simulink library "xrbsDSP_r3"  (Simulink 5.0)
undefined symbols (not defined in the file or in its folder): FIR1, Ft, mem
libraries: xbsIndex_r3 x329
(part 2 of 4)

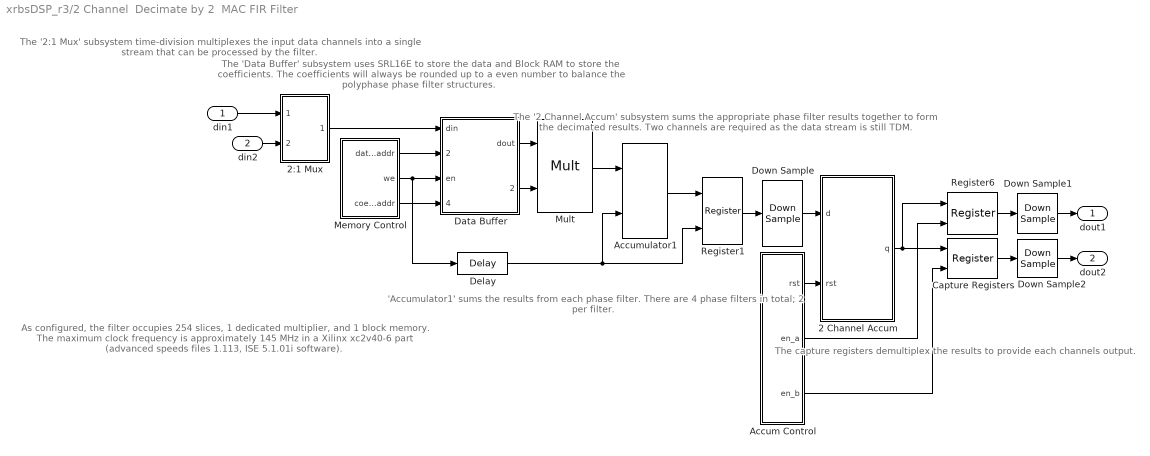
== system xrbsDSP_r3/2 Channel  Decimate by 2  MAC FIR Filter ==
  note: As configured, the  filter occupies 254 slices, 1 dedicated multiplier, and
      | 1 block memory.  The maximum clock frequency is approximately
      | 145 MHz in a Xilinx xc2v40-6 part (advanced speeds files 1.113, ISE
      | 5.1.01i software).
  note: The capture registers demultiplex
      | the results to provide each
      | channels output.
  note: The '2 Channel Accum' subsystem sums the
      | appropriate phase filter results together to
      | form the decimated results.  Two channels
      | are required as the data stream is still TDM.
  note: 'Accumulator1' sums the results
      | from each phase filter.  There
      | are 4 phase filters in total; 2 per
      | filter.
  note: The 'Data Buffer' subsystem uses SRL16E to store
      | the data and Block RAM to store the
      | coefficients. The coefficients will always
      | be rounded up to a even number to balance the
      | polyphase phase filter structures.
  note: The '2:1 Mux' subsystem time-division
      | multiplexes the input data channels
      | into a single stream that can be
      | processed by the filter.
  din1 : Inport
  din2 : Inport  Port=2
  2 Channel Accum : Subsystem
  2:1 Mux : Subsystem
  Accum Control : Subsystem
  Accumulator1 : xbsIndex_r3/Accumulator  n_bits=accum2_bit_width  overflow=Wrap  operation=Add  scale=1  explicit_period=off  period=1  rst=on  hasbypass=on  en=off  dbl_ovrd=off  show_param=off  gen_core=on  use_rpm=off
      settings: xl_area=[0, 0, 0, 0, 0, 0, 0]
  Capture Registers : xbsIndex_r3/Register  init=0  reg_only_valid=off  explicit_period=off  period=1  rst=off  en=on  out_en=on  dbl_ovrd=off  show_param=off
      settings: xl_area=[0, 0, 0, 0, 0, 0, 0]
  Data Buffer : Subsystem
  Delay : xbsIndex_r3/Delay  latency=4  reg_retiming=off  explicit_period=off  period=1  en=off  accept_only_valid=off  init_zero=on  dbl_ovrd=off  show_param=off
      settings: xl_area=[0, 0, 0, 0, 0, 0, 0]
  Down Sample : xbsIndex_r3/Down Sample  sample_ratio=length(coef)/4  sample_phase="Last Value of Frame  (most efficient)"  latency=1  en=off  dbl_ovrd=off  show_param=off
      settings: xl_area=[0, 0, 0, 0, 0, 0, 0]
  Down Sample1 : xbsIndex_r3/Down Sample  sample_ratio=4  sample_phase="Last Value of Frame  (most efficient)"  latency=1  en=off  dbl_ovrd=off  show_param=off
      settings: xl_area=[19 37 0 0 0 0 0]
  Down Sample2 : xbsIndex_r3/Down Sample  sample_ratio=4  sample_phase="Last Value of Frame  (most efficient)"  latency=1  en=off  dbl_ovrd=off  show_param=off
      settings: xl_area=[19 37 0 0 0 0 0]
  Memory Control : Subsystem
  Mult : xbsIndex_r3/Mult  precision=Full  arith_type="Signed  (2's comp)"  n_bits=8  bin_pt=2  quantization=Truncate  overflow=Wrap  latency=2  explicit_period=off  period=1  en=off  dbl_ovrd=off  show_param=off  mult_type=Parallel  oversample=2  use_embedded=on  pipeline=on  use_rpm=off  placement_style=Rectangular Shape  gen_core=on
      settings: xl_area=[0, 0, 0, 0, 0, 0, 0]
  Register1 : xbsIndex_r3/Register  init=0  reg_only_valid=off  explicit_period=off  period=1  rst=off  en=on  out_en=off  dbl_ovrd=off  show_param=off
      settings: xl_area=[0, 0, 0, 0, 0, 0, 0]
  Register6 : xbsIndex_r3/Register  init=0  reg_only_valid=off  explicit_period=off  period=1  rst=off  en=on  out_en=on  dbl_ovrd=off  show_param=off
      settings: xl_area=[0, 0, 0, 0, 0, 0, 0]
  dout1 : Outport
  dout2 : Outport  Port=2
  wires:
  Down Sample2/1 -> dout2/1
  Down Sample1/1 -> dout1/1
  Down Sample/1 -> 2 Channel Accum/1(d)
  din2/1 -> 2:1 Mux/2(din2)
  Accum Control/3(en_b) -> Capture Registers/2
  Accum Control/2(en_a) -> Register6/2
  Accum Control/1(rst) -> 2 Channel Accum/2(rst)
  Capture Registers/1 -> Down Sample2/1
  2 Channel Accum/1(q) -> Register6/1, Capture Registers/1
  Register6/1 -> Down Sample1/1
  Accumulator1/1 -> Register1/1
  Memory Control/3(coef_addr) -> Data Buffer/4(coef_addr)
  Memory Control/2(we) -> Delay/1, Data Buffer/3(en)
  Memory Control/1(data_addr) -> Data Buffer/2(data_addr)
  Data Buffer/1(dout) -> Mult/1
  Mult/1 -> Accumulator1/1
  Delay/1 -> Accumulator1/2, Register1/2
  Register1/1 -> Down Sample/1
  Data Buffer/2(coef_out) -> Mult/2
  2:1 Mux/1(dout) -> Data Buffer/1(din)
  din1/1 -> 2:1 Mux/1(din1)

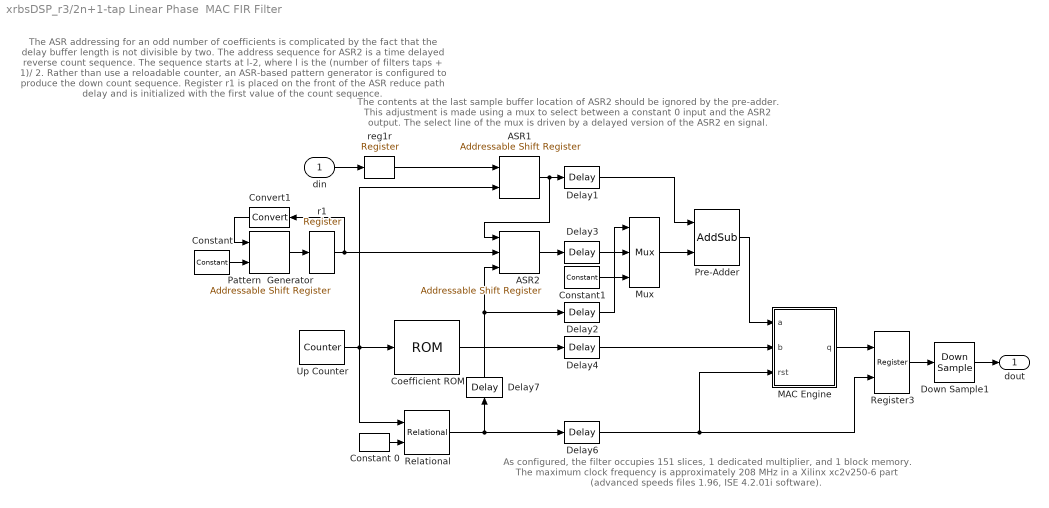
== system xrbsDSP_r3/2n+1-tap Linear Phase  MAC FIR Filter ==
  note: The ASR addressing for an odd number of coefficients is
      | complicated by the fact that the delay buffer length is not
      | divisible by two.  The address sequence for ASR2 is a time
      | delayed reverse count sequence.  The sequence starts at
      | l-2,  where l is the (number of filters taps + 1)/ 2.  Rather
      | than use a reloadable counter, an ASR-based pattern
      | generator is configured to produce the down count
      | sequence.  Register r1 is placed on the front of the ASR
      | reduce path delay and is initialized with the first value of
      | the count sequence.
  note: The contents at the last sample buffer location
      | of ASR2 should be ignored by the pre-adder.
      | This adjustment is made using a mux to select
      | between a constant 0 input and the ASR2 output.
      | The select line of the mux is driven by a delayed
      | version of the ASR2 en signal.
  note: As configured, the  filter occupies 151 slices, 1 dedicated multiplier, and
      | 1 block memory.  The maximum clock frequency is approximately
      | 208 MHz in a Xilinx xc2v250-6 part (advanced speeds files 1.96, ISE
      | 4.2.01i software).
  din : Inport
  ASR1 : xbsIndex_r3/Addressable Shift Register  infer_latency=on  depth=2  initVector=0  explicit_period=off  period=1  accept_only_valid=off  en=off  dbl_ovrd=off  show_param=off  use_rpm=off  gen_core=off
      settings: xl_area=[0, 0, 0, 0, 0, 0, 0]
  ASR2 : xbsIndex_r3/Addressable Shift Register  infer_latency=on  depth=2  initVector=0  explicit_period=off  period=1  accept_only_valid=off  en=on  dbl_ovrd=off  show_param=off  use_rpm=off  gen_core=off
      settings: xl_area=[0, 0, 0, 0, 0, 0, 0]
  Coefficient ROM : xbsIndex_r3/ROM  depth=(length(coef)+1)/2  initVector=coef(1:((length(coef)+1)/2))  arith_type="Signed  (2's comp)"  n_bits=coef_n_bits  bin_pt=coef_bin_pt  latency=1  init_zero=on  explicit_period=off  period=1  rst=off  init_reg=0  en=off  dbl_ovrd=off  show_param=off  distributed_mem=off  use_rpm=off  gen_core=on
      settings: xl_area=[0, 0, 0, 0, 0, 0, 0]
  Constant : xbsIndex_r3/Constant  const=(length(coef)+1)/2-2  arith_type=Unsigned  n_bits=ceil(log2(((length(coef)+1)/2-1)))  bin_pt=0  explicit_period=on  period=smpl_period/((length(coef)+1)/2)  dbl_ovrd=off
  Constant 0 : xbsIndex_r3/Constant  const=0  arith_type=Unsigned  n_bits=1  bin_pt=0  explicit_period=off  period=1  dbl_ovrd=off
  Constant1 : xbsIndex_r3/Constant  const=0  arith_type=Unsigned  n_bits=1  bin_pt=0  explicit_period=off  period=1  dbl_ovrd=off
  Convert1 : xbsIndex_r3/Convert  Orientation=left  arith_type=Unsigned  n_bits=ceil(log2((length(coef)+1)/2))  bin_pt=0  quantization=Truncate  overflow=Wrap  latency=0  explicit_period=off  period=1  dbl_ovrd=off  show_param=off  inserted_by_tool=off
      settings: xl_area=[0, 0, 0, 0, 0, 0, 0]
  Delay1 : xbsIndex_r3/Delay  latency=2  reg_retiming=off  explicit_period=off  period=1  en=off  accept_only_valid=off  init_zero=on  dbl_ovrd=off  show_param=off
      settings: xl_area=[0, 0, 0, 0, 0, 0, 0]
  Delay2 : xbsIndex_r3/Delay  latency=1  reg_retiming=off  explicit_period=off  period=1  en=off  accept_only_valid=off  init_zero=on  dbl_ovrd=off  show_param=off
      settings: xl_area=[0, 0, 0, 0, 0, 0, 0]
  Delay3 : xbsIndex_r3/Delay  latency=1  reg_retiming=off  explicit_period=off  period=1  en=off  accept_only_valid=off  init_zero=on  dbl_ovrd=off  show_param=off
      settings: xl_area=[0, 0, 0, 0, 0, 0, 0]
  Delay4 : xbsIndex_r3/Delay  latency=2  reg_retiming=off  explicit_period=off  period=1  en=off  accept_only_valid=off  init_zero=on  dbl_ovrd=off  show_param=off
      settings: xl_area=[0, 0, 0, 0, 0, 0, 0]
  Delay6 : xbsIndex_r3/Delay  latency=4  reg_retiming=off  explicit_period=off  period=1  en=off  accept_only_valid=off  init_zero=on  dbl_ovrd=off  show_param=off
      settings: xl_area=[0, 0, 0, 0, 0, 0, 0]
  Delay7 : xbsIndex_r3/Delay  Orientation=up  latency=((length(coef)+1)/2)-2  reg_retiming=off  explicit_period=off  period=1  en=off  accept_only_valid=off  init_zero=on  dbl_ovrd=off  show_param=off
      settings: xl_area=[0, 0, 0, 0, 0, 0, 0]
  Down Sample1 : xbsIndex_r3/Down Sample  sample_ratio=(length(coef)+1)/2  sample_phase="Last Value of Frame  (most efficient)"  latency=1  en=off  dbl_ovrd=off  show_param=off
      settings: xl_area=[0, 0, 0, 0, 0, 0, 0]
  MAC Engine : Subsystem
  Mux : xbsIndex_r3/Mux  inputs=2  precision=Full  arith_type="Signed  (2's comp)"  n_bits=8  bin_pt=2  quantization=Truncate  overflow=Wrap  latency=1  explicit_period=off  period=1  en=off  dbl_ovrd=off  show_param=off  mux_type=off  use_rpm=off  gen_core=on
      settings: xl_area=[0, 0, 0, 0, 0, 0, 0]
  Pattern  Generator : xbsIndex_r3/Addressable Shift Register  infer_latency=on  depth=2  initVector=[((length(coef)+1)/2)-1 (0:(length(coef)+1)/2-3)]  explicit_period=off  period=1  accept_only_valid=off  en=off  dbl_ovrd=off  show_param=off  use_rpm=off  gen_core=off
      settings: xl_area=[0, 0, 0, 0, 0, 0, 0]
  Pre-Adder : xbsIndex_r3/AddSub  mode=Addition  precision=Full  arith_type=Unsigned  n_bits=8  bin_pt=2  quantization=Truncate  overflow=Wrap  latency=1  explicit_period=off  period=1  use_carryin=off  use_carryout=off  en=off  dbl_ovrd=off  show_param=off  use_core=on  pipeline=off  use_rpm=off  gen_core=on
      settings: xl_area=[0, 0, 0, 0, 0, 0, 0]
  Register3 : xbsIndex_r3/Register  init=0  reg_only_valid=on  explicit_period=off  period=1  rst=off  en=on  out_en=off  dbl_ovrd=off  show_param=off
      settings: xl_area=[0, 0, 0, 0, 0, 0, 0]
  Relational : xbsIndex_r3/Relational  mode=a=b  latency=1  explicit_period=off  period=1  en=off  dbl_ovrd=off  show_param=off
      settings: xl_area=[0, 0, 0, 0, 0, 0, 0]
  Up Counter : xbsIndex_r3/Counter  cnt_type=Count Limited  n_bits=ceil(log2((length(coef)+1)/2))  bin_pt=0  arith_type=Unsigned  start_count=0  cnt_to=((length(coef)+1)/2)-1  cnt_by_val=1  operation=Up  explicit_period=on  period=smpl_period/((length(coef)+1)/2)  load_pin=off  rst=off  en=off  dbl_ovrd=off  show_param=off  use_rpm=on  gen_core=on
      settings: xl_area=[0, 0, 0, 0, 0, 0, 0]
  r1 : xbsIndex_r3/Register  init=((length(coef)+1)/2)-2  reg_only_valid=off  explicit_period=on  period=smpl_period/((length(coef)+1)/2)  rst=off  en=off  out_en=off  dbl_ovrd=off  show_param=off
      settings: xl_area=[0, 0, 0, 0, 0, 0, 0]
  reg1r : xbsIndex_r3/Register  init=0  reg_only_valid=on  explicit_period=off  period=1  rst=off  en=off  out_en=off  dbl_ovrd=off  show_param=off
      settings: xl_area=[0, 0, 0, 0, 0, 0, 0]
  dout : Outport
  wires:
  Coefficient ROM/1 -> Delay4/1
  Relational/1 -> Delay6/1, Delay7/1
  Constant 0/1 -> Relational/2
  Down Sample1/1 -> dout/1
  din/1 -> reg1r/1
  Up Counter/1 -> Relational/1, Coefficient ROM/1, ASR1/2
  ASR1/1 -> ASR2/1, Delay1/1
  reg1r/1 -> ASR1/1
  Delay1/1 -> Pre-Adder/1
  MAC Engine/1(q) -> Register3/1
  Register3/1 -> Down Sample1/1
  Pre-Adder/1 -> MAC Engine/1(a)
  Delay4/1 -> MAC Engine/2(b)
  Delay6/1 -> Register3/2, MAC Engine/3(rst)
  ASR2/1 -> Delay3/1
  Delay3/1 -> Mux/2
  Pattern  Generator/1 -> r1/1
  Constant/1 -> Pattern  Generator/2
  Convert1/1 -> Pattern  Generator/1
  Mux/1 -> Pre-Adder/2
  Constant1/1 -> Mux/3
  r1/1 -> ASR2/2, Convert1/1
  Delay7/1 -> Delay2/1, ASR2/3
  Delay2/1 -> Mux/1

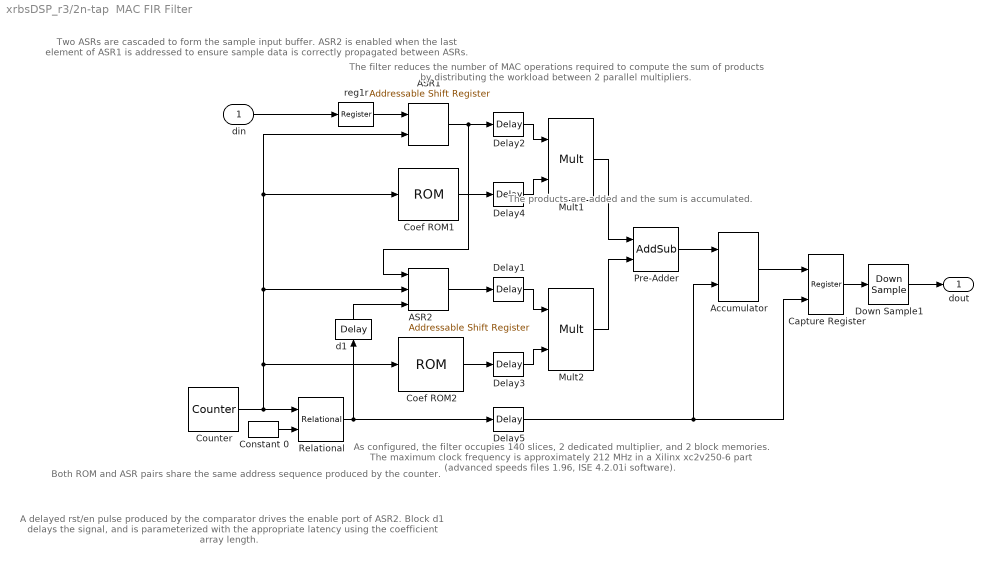
== system xrbsDSP_r3/2n-tap  MAC FIR Filter ==
  note: The filter reduces the number of MAC operations required
      | to compute the sum of products by distributing the workload
      | between 2 parallel multipliers.
  note: Both ROM and ASR pairs share the same
      | address sequence produced by the counter.
  note: The products are added and
      | the sum is accumulated.
  note: As configured, the  filter occupies 140 slices, 2 dedicated multiplier, and
      | 2 block memories.  The maximum clock frequency is approximately
      | 212 MHz in a Xilinx xc2v250-6 part (advanced speeds files 1.96, ISE
      | 4.2.01i software).
  note: Two ASRs are cascaded to form the sample
      | input  buffer.  ASR2 is enabled when the last
      | element of ASR1 is addressed to ensure sample
      | data is correctly propagated between ASRs.
  note: A delayed rst/en pulse produced by the comparator
      | drives the enable port of ASR2.  Block d1 delays the
      | signal, and is parameterized with the appropriate
      | latency using the coefficient array length.
  din : Inport
  ASR1 : xbsIndex_r3/Addressable Shift Register  infer_latency=on  depth=2  initVector=0  explicit_period=off  period=1  accept_only_valid=off  en=off  dbl_ovrd=off  show_param=off  use_rpm=off  gen_core=off
      settings: xl_area=[0, 0, 0, 0, 0, 0, 0]
  ASR2 : xbsIndex_r3/Addressable Shift Register  infer_latency=on  depth=2  initVector=0  explicit_period=off  period=1  accept_only_valid=off  en=on  dbl_ovrd=off  show_param=off  use_rpm=off  gen_core=off
      settings: xl_area=[0, 0, 0, 0, 0, 0, 0]
  Accumulator : xbsIndex_r3/Accumulator  n_bits=ceil(log2(max(1,sum(abs(coef*2^coef_bin_pt)))))+smpl_n_bits + 1  overflow=Wrap  operation=Add  scale=1  explicit_period=off  period=1  rst=on  hasbypass=on  en=off  dbl_ovrd=off  show_param=off  gen_core=on  use_rpm=off
      settings: xl_area=[0, 0, 0, 0, 0, 0, 0]
  Capture Register : xbsIndex_r3/Register  init=0  reg_only_valid=on  explicit_period=off  period=1  rst=off  en=on  out_en=off  dbl_ovrd=off  show_param=off
      settings: xl_area=[0, 0, 0, 0, 0, 0, 0]
  Coef ROM1 : xbsIndex_r3/ROM  depth=length(coef)/2  initVector=coef(1:(length(coef)/2))  arith_type="Signed  (2's comp)"  n_bits=coef_n_bits  bin_pt=coef_bin_pt  latency=1  init_zero=on  explicit_period=off  period=1  rst=off  init_reg=0  en=off  dbl_ovrd=off  show_param=off  distributed_mem=off  use_rpm=off  gen_core=on
      settings: xl_area=[0, 0, 0, 0, 0, 0, 0]
  Coef ROM2 : xbsIndex_r3/ROM  depth=length(coef)/2  initVector=coef((length(coef)/2)+1:length(coef))  arith_type="Signed  (2's comp)"  n_bits=coef_n_bits  bin_pt=coef_bin_pt  latency=1  init_zero=on  explicit_period=off  period=1  rst=off  init_reg=0  en=off  dbl_ovrd=off  show_param=off  distributed_mem=off  use_rpm=off  gen_core=on
      settings: xl_area=[0, 0, 0, 0, 0, 0, 0]
  Constant 0 : xbsIndex_r3/Constant  const=0  arith_type=Unsigned  n_bits=1  bin_pt=0  explicit_period=off  period=1  dbl_ovrd=off
  Counter : xbsIndex_r3/Counter  cnt_type=Count Limited  n_bits=ceil(log2(length(coef)/2))  bin_pt=0  arith_type=Unsigned  start_count=0  cnt_to=(length(coef)/2)-1  cnt_by_val=1  operation=Up  explicit_period=off  period=smpl_period/(length(coef)/2)  load_pin=off  rst=off  en=off  dbl_ovrd=off  show_param=off  use_rpm=on  gen_core=on
      settings: xl_area=[0, 0, 0, 0, 0, 0, 0]
  Delay1 : xbsIndex_r3/Delay  latency=2  reg_retiming=off  explicit_period=off  period=1  en=off  accept_only_valid=off  init_zero=on  dbl_ovrd=off  show_param=off
      settings: xl_area=[0, 0, 0, 0, 0, 0, 0]
  Delay2 : xbsIndex_r3/Delay  latency=2  reg_retiming=off  explicit_period=off  period=1  en=off  accept_only_valid=off  init_zero=on  dbl_ovrd=off  show_param=off
      settings: xl_area=[0, 0, 0, 0, 0, 0, 0]
  Delay3 : xbsIndex_r3/Delay  latency=1  reg_retiming=off  explicit_period=off  period=1  en=off  accept_only_valid=off  init_zero=on  dbl_ovrd=off  show_param=off
      settings: xl_area=[0, 0, 0, 0, 0, 0, 0]
  Delay4 : xbsIndex_r3/Delay  latency=1  reg_retiming=off  explicit_period=off  period=1  en=off  accept_only_valid=off  init_zero=on  dbl_ovrd=off  show_param=off
      settings: xl_area=[0, 0, 0, 0, 0, 0, 0]
  Delay5 : xbsIndex_r3/Delay  latency=4  reg_retiming=off  explicit_period=off  period=1  en=off  accept_only_valid=off  init_zero=on  dbl_ovrd=off  show_param=off
      settings: xl_area=[0, 0, 0, 0, 0, 0, 0]
  Down Sample1 : xbsIndex_r3/Down Sample  sample_ratio=length(coef)/2  sample_phase="Last Value of Frame  (most efficient)"  latency=1  en=off  dbl_ovrd=off  show_param=off
      settings: xl_area=[0, 0, 0, 0, 0, 0, 0]
  Mult1 : xbsIndex_r3/Mult  precision=User Defined  arith_type="Signed  (2's comp)"  n_bits=max(ceil(log2(max(1,max(abs(coef*2^coef_bin_pt)))))+smpl_n_bits + 1,smpl_bin_pt+coef_bin_pt)  bin_pt=smpl_bin_pt+coef_bin_pt  quantization=Truncate  overflow=Wrap  latency=2  explicit_period=off  period=1  en=off  dbl_ovrd=off  show_param=off  mult_type=Parallel  oversample=2  use_embedded=on  pipeline=on  use_rpm=on  placement_style=Rectangular Shape  gen_core=on
      settings: xl_area=[0, 0, 0, 0, 0, 0, 0]
  Mult2 : xbsIndex_r3/Mult  precision=User Defined  arith_type="Signed  (2's comp)"  n_bits=max(ceil(log2(max(1,max(abs(coef*2^coef_bin_pt)))))+smpl_n_bits + 1,smpl_bin_pt+coef_bin_pt)  bin_pt=smpl_bin_pt+coef_bin_pt  quantization=Truncate  overflow=Wrap  latency=2  explicit_period=off  period=1  en=off  dbl_ovrd=off  show_param=off  mult_type=Parallel  oversample=2  use_embedded=on  pipeline=on  use_rpm=on  placement_style=Rectangular Shape  gen_core=on
      settings: xl_area=[0, 0, 0, 0, 0, 0, 0]
  Pre-Adder : xbsIndex_r3/AddSub  mode=Addition  precision=Full  arith_type=Unsigned  n_bits=8  bin_pt=2  quantization=Truncate  overflow=Wrap  latency=1  explicit_period=off  period=1  use_carryin=off  use_carryout=off  en=off  dbl_ovrd=off  show_param=off  use_core=on  pipeline=off  use_rpm=off  gen_core=on
      settings: xl_area=[0, 0, 0, 0, 0, 0, 0]
  Relational : xbsIndex_r3/Relational  mode=a=b  latency=1  explicit_period=off  period=1  en=off  dbl_ovrd=off  show_param=off
      settings: xl_area=[0, 0, 0, 0, 0, 0, 0]
  d1 : xbsIndex_r3/Delay  Orientation=up  latency=(length(coef)/2)-2  reg_retiming=off  explicit_period=off  period=1  en=off  accept_only_valid=off  init_zero=on  dbl_ovrd=off  show_param=off
      settings: xl_area=[0, 0, 0, 0, 0, 0, 0]
  reg1r : xbsIndex_r3/Register  init=0  reg_only_valid=on  explicit_period=off  period=1  rst=off  en=off  out_en=off  dbl_ovrd=off  show_param=off
      settings: xl_area=[0, 0, 0, 0, 0, 0, 0]
  dout : Outport
  wires:
  Constant 0/1 -> Relational/2
  din/1 -> reg1r/1
  reg1r/1 -> ASR1/1
  Coef ROM1/1 -> Delay4/1
  ASR1/1 -> Delay2/1, ASR2/1
  ASR2/1 -> Delay1/1
  Counter/1 -> Relational/1, Coef ROM2/1, ASR2/2, ASR1/2, Coef ROM1/1
  Relational/1 -> d1/1, Delay5/1
  d1/1 -> ASR2/3
  Delay4/1 -> Mult1/2
  Delay2/1 -> Mult1/1
  Delay3/1 -> Mult2/2
  Delay1/1 -> Mult2/1
  Mult2/1 -> Pre-Adder/2
  Mult1/1 -> Pre-Adder/1
  Pre-Adder/1 -> Accumulator/1
  Delay5/1 -> Accumulator/2, Capture Register/2
  Accumulator/1 -> Capture Register/1
  Capture Register/1 -> Down Sample1/1
  Down Sample1/1 -> dout/1
  Coef ROM2/1 -> Delay3/1

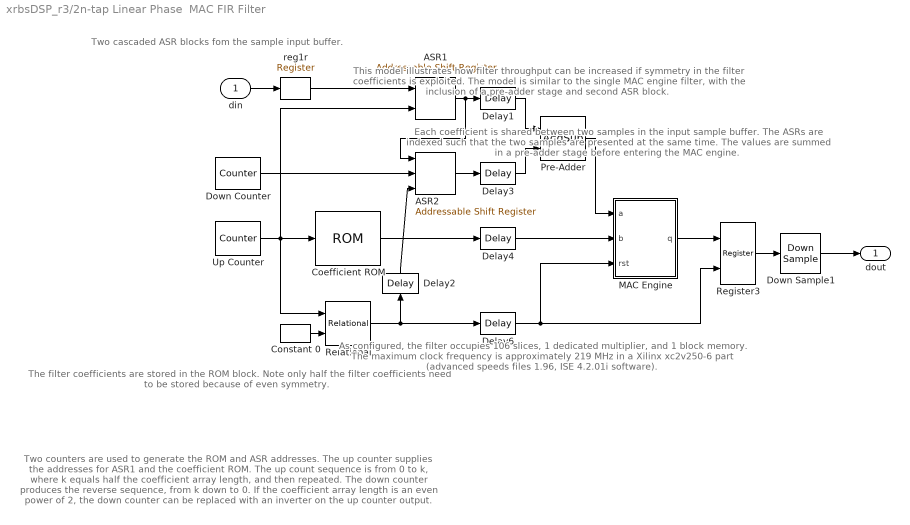
== system xrbsDSP_r3/2n-tap Linear Phase  MAC FIR Filter ==
  note: Each coefficient is shared between two samples
      | in the input sample buffer.   The ASRs are indexed
      | such that the two samples are presented at the same
      | time.  The values are summed in a pre-adder stage
      | before entering the MAC engine.
  note: Two cascaded ASR blocks fom the sample input buffer.
  note: Two counters are used to generate the ROM and ASR
      | addresses.  The up counter supplies the addresses
      | for ASR1 and the coefficient ROM.  The up count
      | sequence is from 0 to k, where k equals half the
      | coefficient array length, and then repeated.  The
      | down counter produces the reverse sequence, from
      | k down to 0.  If the coefficient array length is an even
      | power of 2, the down counter can be replaced with
      | an inverter on the up counter output.
  note: The filter coefficients are stored in the ROM block.
      | Note only half the filter coefficients need to be
      | stored because of even symmetry.
  note: As configured, the  filter occupies 106 slices, 1 dedicated multiplier, and
      | 1 block memory.  The maximum clock frequency is approximately
      | 219 MHz in a Xilinx xc2v250-6 part (advanced speeds files 1.96, ISE
      | 4.2.01i software).
  note: This model illustrates how filter throughput can be
      | increased if symmetry in the filter coefficients is
      | exploited.  The model is similar to the single MAC
      | engine filter, with the inclusion of a pre-adder stage
      | and second ASR block.
  din : Inport
  ASR1 : xbsIndex_r3/Addressable Shift Register  infer_latency=on  depth=2  initVector=0  explicit_period=off  period=1  accept_only_valid=off  en=off  dbl_ovrd=off  show_param=off  use_rpm=off  gen_core=off
      settings: xl_area=[0, 0, 0, 0, 0, 0, 0]
  ASR2 : xbsIndex_r3/Addressable Shift Register  infer_latency=on  depth=2  initVector=0  explicit_period=off  period=1  accept_only_valid=off  en=on  dbl_ovrd=off  show_param=off  use_rpm=off  gen_core=off
      settings: xl_area=[0, 0, 0, 0, 0, 0, 0]
  Coefficient ROM : xbsIndex_r3/ROM  depth=length(coef)/2  initVector=coef(1:(length(coef)/2))  arith_type="Signed  (2's comp)"  n_bits=coef_n_bits  bin_pt=coef_bin_pt  latency=1  init_zero=on  explicit_period=off  period=1  rst=off  init_reg=0  en=off  dbl_ovrd=off  show_param=off  distributed_mem=off  use_rpm=off  gen_core=on
      settings: xl_area=[0, 0, 0, 0, 0, 0, 0]
  Constant 0 : xbsIndex_r3/Constant  const=0  arith_type=Unsigned  n_bits=1  bin_pt=0  explicit_period=off  period=1  dbl_ovrd=off
  Delay1 : xbsIndex_r3/Delay  latency=1  reg_retiming=off  explicit_period=off  period=1  en=off  accept_only_valid=off  init_zero=on  dbl_ovrd=off  show_param=off
      settings: xl_area=[0, 0, 0, 0, 0, 0, 0]
  Delay2 : xbsIndex_r3/Delay  Orientation=up  latency=(length(coef)/2)-2  reg_retiming=off  explicit_period=off  period=1  en=off  accept_only_valid=off  init_zero=on  dbl_ovrd=off  show_param=off
      settings: xl_area=[0, 0, 0, 0, 0, 0, 0]
  Delay3 : xbsIndex_r3/Delay  latency=1  reg_retiming=off  explicit_period=off  period=1  en=off  accept_only_valid=off  init_zero=on  dbl_ovrd=off  show_param=off
      settings: xl_area=[0, 0, 0, 0, 0, 0, 0]
  Delay4 : xbsIndex_r3/Delay  latency=1  reg_retiming=off  explicit_period=off  period=1  en=off  accept_only_valid=off  init_zero=on  dbl_ovrd=off  show_param=off
      settings: xl_area=[0, 0, 0, 0, 0, 0, 0]
  Delay6 : xbsIndex_r3/Delay  latency=3  reg_retiming=off  explicit_period=off  period=1  en=off  accept_only_valid=off  init_zero=on  dbl_ovrd=off  show_param=off
      settings: xl_area=[0, 0, 0, 0, 0, 0, 0]
  Down Counter : xbsIndex_r3/Counter  cnt_type=Count Limited  n_bits=ceil(log2(length(coef)/2))  bin_pt=0  arith_type=Unsigned  start_count=(length(coef)/2)-1  cnt_to=0  cnt_by_val=1  operation=Down  explicit_period=on  period=smpl_period/(length(coef)/2)  load_pin=off  rst=off  en=off  dbl_ovrd=off  show_param=off  use_rpm=on  gen_core=on
      settings: xl_area=[0, 0, 0, 0, 0, 0, 0]
  Down Sample1 : xbsIndex_r3/Down Sample  sample_ratio=length(coef)/2  sample_phase="Last Value of Frame  (most efficient)"  latency=1  en=off  dbl_ovrd=off  show_param=off
      settings: xl_area=[0, 0, 0, 0, 0, 0, 0]
  MAC Engine : Subsystem
  Pre-Adder : xbsIndex_r3/AddSub  mode=Addition  precision=Full  arith_type=Unsigned  n_bits=8  bin_pt=2  quantization=Truncate  overflow=Wrap  latency=1  explicit_period=off  period=1  use_carryin=off  use_carryout=off  en=off  dbl_ovrd=off  show_param=off  use_core=on  pipeline=off  use_rpm=off  gen_core=on
      settings: xl_area=[0, 0, 0, 0, 0, 0, 0]
  Register3 : xbsIndex_r3/Register  init=0  reg_only_valid=on  explicit_period=off  period=1  rst=off  en=on  out_en=off  dbl_ovrd=off  show_param=off
      settings: xl_area=[0, 0, 0, 0, 0, 0, 0]
  Relational : xbsIndex_r3/Relational  mode=a=b  latency=1  explicit_period=off  period=1  en=off  dbl_ovrd=off  show_param=off
      settings: xl_area=[0, 0, 0, 0, 0, 0, 0]
  Up Counter : xbsIndex_r3/Counter  cnt_type=Count Limited  n_bits=ceil(log2(length(coef)/2))  bin_pt=0  arith_type=Unsigned  start_count=0  cnt_to=(length(coef)/2)-1  cnt_by_val=1  operation=Up  explicit_period=on  period=smpl_period/(length(coef)/2)  load_pin=off  rst=off  en=off  dbl_ovrd=off  show_param=off  use_rpm=on  gen_core=on
      settings: xl_area=[0, 0, 0, 0, 0, 0, 0]
  reg1r : xbsIndex_r3/Register  init=0  reg_only_valid=on  explicit_period=off  period=1  rst=off  en=off  out_en=off  dbl_ovrd=off  show_param=off
      settings: xl_area=[0, 0, 0, 0, 0, 0, 0]
  dout : Outport
  wires:
  Coefficient ROM/1 -> Delay4/1
  Relational/1 -> Delay2/1, Delay6/1
  Constant 0/1 -> Relational/2
  Down Sample1/1 -> dout/1
  din/1 -> reg1r/1
  Up Counter/1 -> Relational/1, Coefficient ROM/1, ASR1/2
  ASR1/1 -> ASR2/1, Delay1/1
  reg1r/1 -> ASR1/1
  Delay1/1 -> Pre-Adder/1
  MAC Engine/1(q) -> Register3/1
  Register3/1 -> Down Sample1/1
  ASR2/1 -> Delay3/1
  Delay3/1 -> Pre-Adder/2
  Pre-Adder/1 -> MAC Engine/1(a)
  Delay2/1 -> ASR2/3
  Delay4/1 -> MAC Engine/2(b)
  Delay6/1 -> Register3/2, MAC Engine/3(rst)
  Down Counter/1 -> ASR2/2

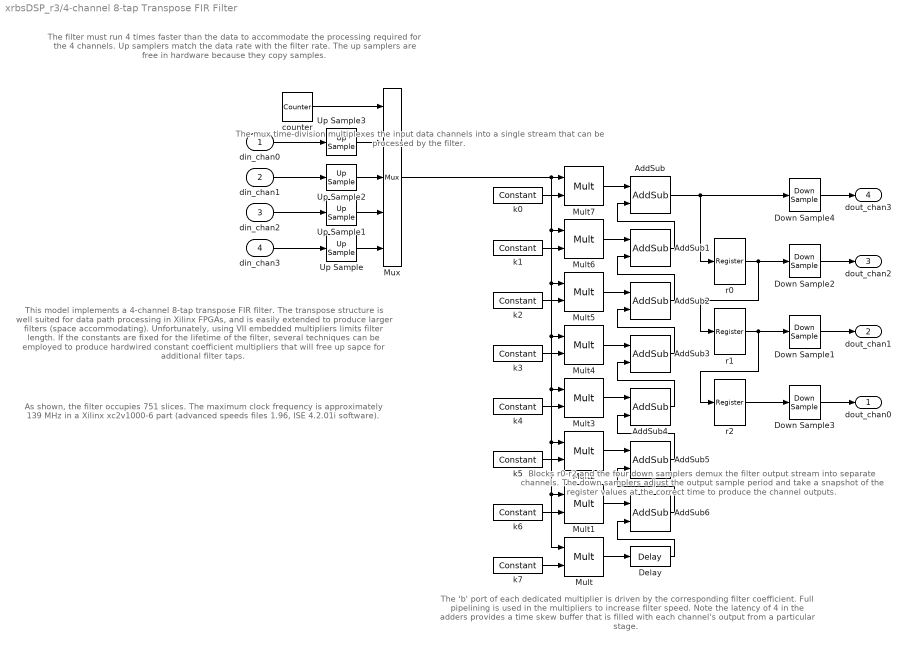
== system xrbsDSP_r3/4-channel 8-tap Transpose FIR Filter ==
  note: This model implements a 4-channel 8-tap transpose FIR filter.
      | The transpose structure is well suited for data path processing
      | in Xilinx FPGAs, and is easily extended to produce larger filters
      | (space accommodating).  Unfortunately, using VII embedded
      | multipliers limits filter length.  If the constants are fixed for the
      | lifetime of the filter, several techniques can be employed to
      | produce hardwired constant coefficient multipliers that will free
      | up sapce for additional filter taps.
  note: Blocks r0-r2 and the four down samplers
      | demux the filter output stream into separate
      | channels.  The down samplers adjust the
      | output sample period and take a snapshot
      | of the register values at the correct time to
      | produce the channel outputs.
  note: The filter must run 4 times faster than the data to
      | accommodate the processing required for the 4
      | channels.  Up samplers match the data
      | rate with the filter rate.  The up samplers are free
      | in hardware because they copy samples.
  note: The mux time-division multiplexes the input data
      | channels into a single stream that can be
      | processed by the filter.
  note: The 'b' port of each dedicated multiplier is driven by the corresponding
      | filter coefficient.  Full pipelining is used in the multipliers to increase
      | filter speed.  Note the latency of 4 in the adders provides a time skew
      | buffer that is filled with each channel's output from a particular stage.
  note: As shown, the  filter occupies 751 slices.  The maximum clock
      | frequency is approximately 139 MHz in a Xilinx xc2v1000-6 part
      | (advanced speeds files 1.96, ISE 4.2.01i software).
  din_chan0 : Inport
  din_chan1 : Inport  Port=2
  din_chan2 : Inport  Port=3
  din_chan3 : Inport  Port=4
  AddSub{,1..6} (7 alike) : xbsIndex_r3/AddSub  mode=Addition  precision=Full  arith_type=Unsigned  n_bits=8  bin_pt=2  quantization=Truncate  overflow=Wrap  latency=4  explicit_period=off  period=1  use_carryin=off  use_carryout=off  en=off  dbl_ovrd=off  show_param=off  use_core=on  pipeline=off  use_rpm=off  gen_core=on
      settings: xl_area=[0, 0, 0, 0, 0, 0, 0]
  Delay : xbsIndex_r3/Delay  latency=4  reg_retiming=off  explicit_period=off  period=1  en=off  accept_only_valid=off  init_zero=off  dbl_ovrd=off  show_param=off
      settings: xl_area=[0, 0, 0, 0, 0, 0, 0]
  Down Sample{1..4} (4 alike) : xbsIndex_r3/Down Sample  sample_ratio=4  sample_phase="Last Value of Frame  (most efficient)"  latency=1  en=off  dbl_ovrd=off  show_param=off
      settings: xl_area=[0, 0, 0, 0, 0, 0, 0]
  Mult{,1..7} (8 alike) : xbsIndex_r3/Mult  precision=Full  arith_type="Signed  (2's comp)"  n_bits=8  bin_pt=2  quantization=Truncate  overflow=Wrap  latency=3  explicit_period=off  period=1  en=off  dbl_ovrd=off  show_param=off  mult_type=Parallel  oversample=2  use_embedded=on  pipeline=on  use_rpm=off  placement_style=Rectangular Shape  gen_core=on
      settings: xl_area=[0, 0, 0, 0, 0, 0, 0]
  Mux : xbsIndex_r3/Mux  inputs=4  precision=Full  arith_type="Signed  (2's comp)"  n_bits=8  bin_pt=2  quantization=Truncate  overflow=Wrap  latency=1  explicit_period=off  period=1  en=off  dbl_ovrd=off  show_param=off  mux_type=off  use_rpm=off  gen_core=on
      settings: xl_area=[0, 0, 0, 0, 0, 0, 0]
  Up Sample{,1..3} (4 alike) : xbsIndex_r3/Up Sample  sample_ratio=4  copy_samples=on  dbl_ovrd=off  show_param=off
      settings: xl_area=[0, 0, 0, 0, 0, 0, 0]
  counter : xbsIndex_r3/Counter  cnt_type=Free Running  n_bits=2  bin_pt=0  arith_type=Unsigned  start_count=0  cnt_to=Inf  cnt_by_val=1  operation=Up  explicit_period=off  period=smpl_period/4  load_pin=off  rst=off  en=off  dbl_ovrd=off  show_param=off  use_rpm=off  gen_core=on
      settings: xl_area=[0, 0, 0, 0, 0, 0, 0]
  k0 : xbsIndex_r3/Constant  const=coef(1)  arith_type="Signed  (2's comp)"  n_bits=coef_n_bits  bin_pt=coef_bin_pt  explicit_period=off  period=1  dbl_ovrd=off
  k1 : xbsIndex_r3/Constant  const=coef(2)  arith_type="Signed  (2's comp)"  n_bits=coef_n_bits  bin_pt=coef_bin_pt  explicit_period=off  period=1  dbl_ovrd=off
  k2 : xbsIndex_r3/Constant  const=coef(3)  arith_type="Signed  (2's comp)"  n_bits=coef_n_bits  bin_pt=coef_bin_pt  explicit_period=off  period=1  dbl_ovrd=off
  k3 : xbsIndex_r3/Constant  const=coef(4)  arith_type="Signed  (2's comp)"  n_bits=coef_n_bits  bin_pt=coef_bin_pt  explicit_period=off  period=1  dbl_ovrd=off
  k4 : xbsIndex_r3/Constant  const=coef(5)  arith_type="Signed  (2's comp)"  n_bits=coef_n_bits  bin_pt=coef_bin_pt  explicit_period=off  period=1  dbl_ovrd=off
  k5 : xbsIndex_r3/Constant  const=coef(6)  arith_type="Signed  (2's comp)"  n_bits=coef_n_bits  bin_pt=coef_bin_pt  explicit_period=off  period=1  dbl_ovrd=off
  k6 : xbsIndex_r3/Constant  const=coef(7)  arith_type="Signed  (2's comp)"  n_bits=coef_n_bits  bin_pt=coef_bin_pt  explicit_period=off  period=1  dbl_ovrd=off
  k7 : xbsIndex_r3/Constant  const=coef(8)  arith_type="Signed  (2's comp)"  n_bits=coef_n_bits  bin_pt=coef_bin_pt  explicit_period=off  period=1  dbl_ovrd=off
  r0 : xbsIndex_r3/Register  init=0  reg_only_valid=off  explicit_period=off  period=1  rst=off  en=off  out_en=off  dbl_ovrd=off  show_param=off
      settings: xl_area=[0, 0, 0, 0, 0, 0, 0]
  r1 : xbsIndex_r3/Register  init=0  reg_only_valid=off  explicit_period=off  period=1  rst=off  en=off  out_en=off  dbl_ovrd=off  show_param=off
      settings: xl_area=[0, 0, 0, 0, 0, 0, 0]
  r2 : xbsIndex_r3/Register  init=0  reg_only_valid=off  explicit_period=off  period=1  rst=off  en=off  out_en=off  dbl_ovrd=off  show_param=off
      settings: xl_area=[0, 0, 0, 0, 0, 0, 0]
  dout_chan0 : Outport
  dout_chan1 : Outport  Port=2
  dout_chan2 : Outport  Port=3
  dout_chan3 : Outport  Port=4
  wires:
  Mux/1 -> Mult7/1, Mult5/1, Mult4/1, Mult3/1, Mult2/1, Mult1/1, Mult/1, Mult6/1
  din_chan0/1 -> Up Sample3/1
  din_chan1/1 -> Up Sample2/1
  din_chan2/1 -> Up Sample1/1
  din_chan3/1 -> Up Sample/1
  counter/1 -> Mux/1
  Up Sample/1 -> Mux/5
  Up Sample1/1 -> Mux/4
  Up Sample2/1 -> Mux/3
  Up Sample3/1 -> Mux/2
  r0/1 -> Down Sample2/1, r1/1
  r1/1 -> Down Sample1/1, r2/1
  r2/1 -> Down Sample3/1
  Down Sample4/1 -> dout_chan3/1
  Down Sample2/1 -> dout_chan2/1
  Down Sample1/1 -> dout_chan1/1
  Down Sample3/1 -> dout_chan0/1
  AddSub/1 -> Down Sample4/1, r0/1
  Mult7/1 -> AddSub/1
  Mult6/1 -> AddSub1/1
  AddSub1/1 -> AddSub/2
  Mult5/1 -> AddSub2/1
  AddSub2/1 -> AddSub1/2
  Mult4/1 -> AddSub3/1
  AddSub3/1 -> AddSub2/2
  Mult3/1 -> AddSub4/1
  AddSub4/1 -> AddSub3/2
  Mult2/1 -> AddSub5/1
  AddSub5/1 -> AddSub4/2
  Mult1/1 -> AddSub6/1
  AddSub6/1 -> AddSub5/2
  Mult/1 -> Delay/1
  Delay/1 -> AddSub6/2
  k7/1 -> Mult/2
  k6/1 -> Mult1/2
  k5/1 -> Mult2/2
  k4/1 -> Mult3/2
  k3/1 -> Mult4/2
  k2/1 -> Mult5/2
  k1/1 -> Mult6/2
  k0/1 -> Mult7/2

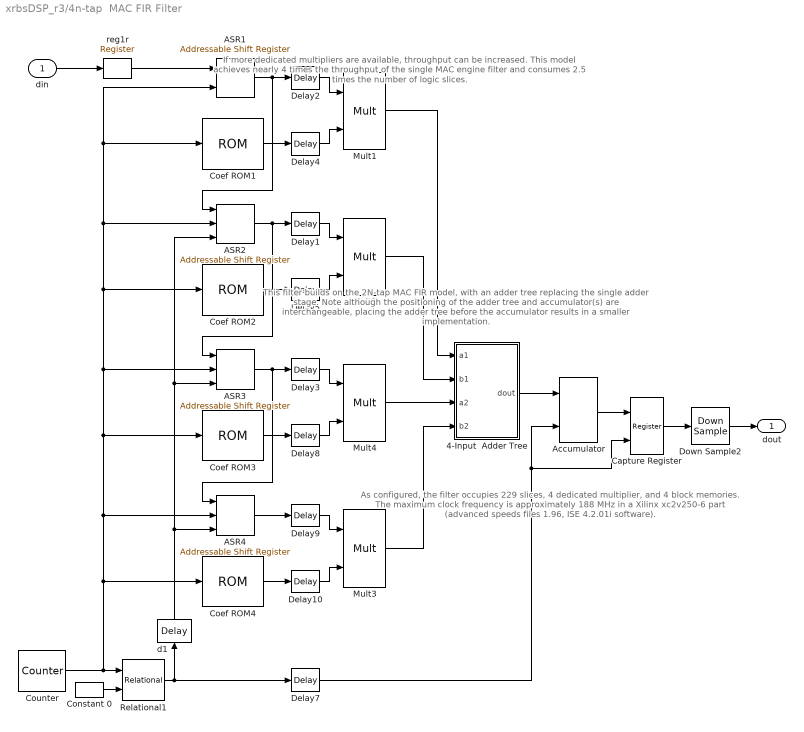
== system xrbsDSP_r3/4n-tap  MAC FIR Filter ==
  note: This filter builds on the 2N-tap MAC FIR model, with an adder tree
      | replacing the single adder stage.  Note although the positioning
      | of the adder tree and accumulator(s) are interchangeable, placing
      | the adder tree before the accumulator results in a smaller
      | implementation.
  note: As configured, the filter occupies 229 slices, 4 dedicated multiplier,
      | and 4 block memories.  The maximum clock frequency is approximately
      | 188 MHz in a Xilinx xc2v250-6 part (advanced speeds files 1.96, ISE
      | 4.2.01i software).
  note: If more dedicated multipliers are available, throughput
      | can be increased.  This model achieves nearly 4 times
      | the throughput of the single MAC engine filter and
      | consumes 2.5 times the number of logic slices.
  din : Inport
  4-Input  Adder Tree : Subsystem
  ASR1 : xbsIndex_r3/Addressable Shift Register  infer_latency=on  depth=2  initVector=0  explicit_period=off  period=1  accept_only_valid=off  en=off  dbl_ovrd=off  show_param=off  use_rpm=off  gen_core=off
      settings: xl_area=[0, 0, 0, 0, 0, 0, 0]
  ASR2 : xbsIndex_r3/Addressable Shift Register  infer_latency=on  depth=2  initVector=0  explicit_period=off  period=1  accept_only_valid=off  en=on  dbl_ovrd=off  show_param=off  use_rpm=off  gen_core=off
      settings: xl_area=[0, 0, 0, 0, 0, 0, 0]
  ASR3 : xbsIndex_r3/Addressable Shift Register  infer_latency=on  depth=2  initVector=0  explicit_period=off  period=1  accept_only_valid=off  en=on  dbl_ovrd=off  show_param=off  use_rpm=off  gen_core=off
      settings: xl_area=[0, 0, 0, 0, 0, 0, 0]
  ASR4 : xbsIndex_r3/Addressable Shift Register  infer_latency=on  depth=2  initVector=0  explicit_period=off  period=1  accept_only_valid=off  en=on  dbl_ovrd=off  show_param=off  use_rpm=off  gen_core=off
      settings: xl_area=[0, 0, 0, 0, 0, 0, 0]
  Accumulator : xbsIndex_r3/Accumulator  n_bits=ceil(log2(max(1,sum(abs(coef*2^coef_bin_pt)))))+smpl_n_bits + 1  overflow=Wrap  operation=Add  scale=1  explicit_period=off  period=1  rst=on  hasbypass=on  en=off  dbl_ovrd=off  show_param=off  gen_core=on  use_rpm=off
      settings: xl_area=[0, 0, 0, 0, 0, 0, 0]
  Capture Register : xbsIndex_r3/Register  init=0  reg_only_valid=on  explicit_period=off  period=1  rst=off  en=on  out_en=off  dbl_ovrd=off  show_param=off
      settings: xl_area=[0, 0, 0, 0, 0, 0, 0]
  Coef ROM1 : xbsIndex_r3/ROM  depth=length(coef)/4  initVector=coef(1:(length(coef)/4))  arith_type="Signed  (2's comp)"  n_bits=coef_n_bits  bin_pt=coef_bin_pt  latency=1  init_zero=on  explicit_period=off  period=1  rst=off  init_reg=0  en=off  dbl_ovrd=off  show_param=off  distributed_mem=off  use_rpm=off  gen_core=on
      settings: xl_area=[0, 0, 0, 0, 0, 0, 0]
  Coef ROM2 : xbsIndex_r3/ROM  depth=length(coef)/4  initVector=coef((length(coef)/4)+1:length(coef)/2)  arith_type="Signed  (2's comp)"  n_bits=coef_n_bits  bin_pt=coef_bin_pt  latency=1  init_zero=on  explicit_period=off  period=1  rst=off  init_reg=0  en=off  dbl_ovrd=off  show_param=off  distributed_mem=off  use_rpm=off  gen_core=on
      settings: xl_area=[0, 0, 0, 0, 0, 0, 0]
  Coef ROM3 : xbsIndex_r3/ROM  depth=length(coef)/4  initVector=coef((length(coef)/2)+1:(3/4)*length(coef))  arith_type="Signed  (2's comp)"  n_bits=coef_n_bits  bin_pt=coef_bin_pt  latency=1  init_zero=on  explicit_period=off  period=1  rst=off  init_reg=0  en=off  dbl_ovrd=off  show_param=off  distributed_mem=off  use_rpm=off  gen_core=on
      settings: xl_area=[0, 0, 0, 0, 0, 0, 0]
  Coef ROM4 : xbsIndex_r3/ROM  depth=length(coef)/4  initVector=coef((3/4)*length(coef)+1:length(coef))  arith_type="Signed  (2's comp)"  n_bits=coef_n_bits  bin_pt=coef_bin_pt  latency=1  init_zero=on  explicit_period=off  period=1  rst=off  init_reg=0  en=off  dbl_ovrd=off  show_param=off  distributed_mem=off  use_rpm=off  gen_core=on
      settings: xl_area=[0, 0, 0, 0, 0, 0, 0]
  Constant 0 : xbsIndex_r3/Constant  const=0  arith_type=Unsigned  n_bits=1  bin_pt=0  explicit_period=off  period=1  dbl_ovrd=off
  Counter : xbsIndex_r3/Counter  cnt_type=Count Limited  n_bits=ceil(log2(length(coef)/4))  bin_pt=0  arith_type=Unsigned  start_count=0  cnt_to=(length(coef)/4)-1  cnt_by_val=1  operation=Up  explicit_period=on  period=smpl_period/(length(coef)/4)  load_pin=off  rst=off  en=off  dbl_ovrd=off  show_param=off  use_rpm=on  gen_core=on
      settings: xl_area=[0, 0, 0, 0, 0, 0, 0]
  Delay{1..3,9} (4 alike) : xbsIndex_r3/Delay  latency=2  reg_retiming=off  explicit_period=off  period=1  en=off  accept_only_valid=off  init_zero=on  dbl_ovrd=off  show_param=off
      settings: xl_area=[0, 0, 0, 0, 0, 0, 0]
  Delay{4..5,8,10} (4 alike) : xbsIndex_r3/Delay  latency=1  reg_retiming=off  explicit_period=off  period=1  en=off  accept_only_valid=off  init_zero=on  dbl_ovrd=off  show_param=off
      settings: xl_area=[0, 0, 0, 0, 0, 0, 0]
  Delay7 : xbsIndex_r3/Delay  latency=5  reg_retiming=off  explicit_period=off  period=1  en=off  accept_only_valid=off  init_zero=on  dbl_ovrd=off  show_param=off
      settings: xl_area=[0, 0, 0, 0, 0, 0, 0]
  Down Sample2 : xbsIndex_r3/Down Sample  sample_ratio=length(coef)/4  sample_phase="Last Value of Frame  (most efficient)"  latency=1  en=off  dbl_ovrd=off  show_param=off
      settings: xl_area=[0, 0, 0, 0, 0, 0, 0]
  Mult{1..4} (4 alike) : xbsIndex_r3/Mult  precision=User Defined  arith_type="Signed  (2's comp)"  n_bits=max(ceil(log2(max(1,max(abs(coef*2^coef_bin_pt)))))+smpl_n_bits + 1,smpl_bin_pt+coef_bin_pt)  bin_pt=smpl_bin_pt+coef_bin_pt  quantization=Truncate  overflow=Wrap  latency=2  explicit_period=off  period=1  en=off  dbl_ovrd=off  show_param=off  mult_type=Parallel  oversample=2  use_embedded=on  pipeline=on  use_rpm=on  placement_style=Rectangular Shape  gen_core=on
      settings: xl_area=[0, 0, 0, 0, 0, 0, 0]
  Relational1 : xbsIndex_r3/Relational  mode=a=b  latency=1  explicit_period=off  period=1  en=off  dbl_ovrd=off  show_param=off
      settings: xl_area=[0, 0, 0, 0, 0, 0, 0]
  d1 : xbsIndex_r3/Delay  Orientation=up  latency=(length(coef)/4)-2  reg_retiming=off  explicit_period=off  period=1  en=off  accept_only_valid=off  init_zero=on  dbl_ovrd=off  show_param=off
      settings: xl_area=[0, 0, 0, 0, 0, 0, 0]
  reg1r : xbsIndex_r3/Register  init=0  reg_only_valid=on  explicit_period=off  period=1  rst=off  en=off  out_en=off  dbl_ovrd=off  show_param=off
      settings: xl_area=[0, 0, 0, 0, 0, 0, 0]
  dout : Outport
  wires:
  Constant 0/1 -> Relational1/2
  din/1 -> reg1r/1
  reg1r/1 -> ASR1/1
  Coef ROM1/1 -> Delay4/1
  ASR1/1 -> Delay2/1, ASR2/1
  Coef ROM2/1 -> Delay5/1
  ASR2/1 -> Delay1/1, ASR3/1
  Delay2/1 -> Mult1/1
  Delay1/1 -> Mult2/1
  Mult1/1 -> 4-Input  Adder Tree/1(a1)
  Mult2/1 -> 4-Input  Adder Tree/2(b1)
  Counter/1 -> Relational1/1, ASR4/2, Coef ROM3/1, ASR3/2, Coef ROM2/1, ASR2/2, ASR1/2, Coef ROM1/1, Coef ROM4/1
  Relational1/1 -> d1/1, Delay7/1
  Coef ROM3/1 -> Delay8/1
  ASR3/1 -> Delay3/1, ASR4/1
  Delay3/1 -> Mult4/1
  Coef ROM4/1 -> Delay10/1
  ASR4/1 -> Delay9/1
  Delay9/1 -> Mult3/1
  Mult3/1 -> 4-Input  Adder Tree/4(b2)
  Delay5/1 -> Mult2/2
  Delay8/1 -> Mult4/2
  Delay4/1 -> Mult1/2
  Delay10/1 -> Mult3/2
  d1/1 -> ASR4/3, ASR2/3, ASR3/3
  Accumulator/1 -> Capture Register/1
  Capture Register/1 -> Down Sample2/1
  Down Sample2/1 -> dout/1
  Mult4/1 -> 4-Input  Adder Tree/3(a2)
  4-Input  Adder Tree/1(dout) -> Accumulator/1
  Delay7/1 -> Accumulator/2, Capture Register/2

== system xrbsDSP_r3/CIC Filter ==
  note: The CIC filter is constructed out of differentiators and integrators and
      | a sample rate change. This block provides a full precision result and is
      | dynamically built given the parameters entered in the dialog box. The
      | dynamic rebuilding script can switch which side the integrators and
      | differentiators are on and also change between an up and down sampler
      | depending on whether an Interpolator or decimator is selected respectively.
      | The number of stages selected control how many integrators and
      | differentiators are used.
  note: The Interpoiation by 48, 4 stage CIC filter occupies 204 slices.
      | The maximum clock frequency is approximately
      | 232 MHz in a Xilinx xc2vp2-7 part (advanced speeds
      | files 1.78, ISE 5.2.03i software).
  In1 : Inport
  Differentiator1 : Subsystem  mask(Differentiator Stage){m=m, output_bitwidth=1 + input_bitwidth, output_binpt=input_binpt}
      mask prompts: m "Differential Delay"; output_bitwidth "Output Bit Width"; output_binpt "Output Binary Point"
      mask help: Multi-Channel Differentiator
  Differentiator2 : Subsystem  mask(Differentiator Stage){m=m, output_bitwidth=2+ input_bitwidth, output_binpt=input_binpt}
      mask prompts: m "Differential Delay"; output_bitwidth "Output Bit Width"; output_binpt "Output Binary Point"
      mask help: Multi-Channel Differentiator
  Differentiator3 : Subsystem  mask(Differentiator Stage){m=m, output_bitwidth=3+ input_bitwidth, output_binpt=input_binpt}
      mask prompts: m "Differential Delay"; output_bitwidth "Output Bit Width"; output_binpt "Output Binary Point"
      mask help: Multi-Channel Differentiator
  Integrator1 : Subsystem  mask(Integrator Stage){output_bitwidth=ceil(log2(2^(2*stages-4)*(rate_change*m)^(4-stages)) + input_bitwidth)}
      mask prompts: output_bitwidth "Output Bit Width"
      mask help: Multi Channel Integrator
  Integrator2 : Subsystem  mask(Integrator Stage){output_bitwidth=ceil(log2(2^(2*stages-5)*(rate_change*m)^(5-stages)) + input_bitwidth)}
      mask prompts: output_bitwidth "Output Bit Width"
      mask help: Multi Channel Integrator
  Integrator3 : Subsystem  mask(Integrator Stage){output_bitwidth=ceil(log2(2^(2*stages-6)*(rate_change*m)^(6-stages)) + input_bitwidth)}
      mask prompts: output_bitwidth "Output Bit Width"
      mask help: Multi Channel Integrator
  Up Sample : xbsIndex_r3/Up Sample  sample_ratio=rate_change  copy_samples=off  dbl_ovrd=off  show_param=off
      settings: xl_area=[0, 0, 0, 0, 0, 0, 0]
  Out1 : Outport
  wires:
  Integrator3/1(Out1) -> Out1/1
  Differentiator3/1(Out1) -> Up Sample/1
  Differentiator2/1(Out1) -> Differentiator3/1(In1)
  Integrator2/1(Out1) -> Integrator3/1(In1)
  Differentiator1/1(Out1) -> Differentiator2/1(In1)
  Integrator1/1(Out1) -> Integrator2/1(In1)
  Up Sample/1 -> Integrator1/1(In1)
  In1/1 -> Differentiator1/1(In1)

== system xrbsDSP_r3/Dual Port Memory Interpolation MAC FIR Filter ==
  note: The control logic provides the
      | necessary address logic for the
      | Dual Port RAM. The control logic
      | creates a cyclic RAM buffer for
      | port A (data buffer) to create the
      | shifting effect required.
  note: A 'Dual Port Block RAM' subystem implements the
      | input data buffer.  The address port runs n times
      | faster than the data port, where n is the number
      | of filter taps.
      |
      | The filter coefficients are also stored in the same
      | Dual Port Block RAM and are output from port B.
  note: As configured, the filter occupies 96 slices,
      | 1 dedicated multiplier, and 1 block memory.
      | The maximum clock frequency is approximately
      | 184 MHz in a Xilinx xc2vp2-7 part (advanced
      | speeds files 1.69, ISE 5.1.01i software).
  note: A capture register is required for streaming
      | operation, since the MAC engine reloads its
      | accumulator with an incoming sample after
      | computing the last partial product for an output
      | sample.
  note: A down sampler reduces the capture register
      | sample period to the output sample period. Note that
      | the down sample is less than the up sample to achieve
      | the correct interpolation rate.
      |
      | The block is configured with latency to obtain  the
      | most efficient hardware implementation.  The down
      | sampling rate is equal to the coefficient array length.
  Din : Inport
  Accumulator : xbsIndex_r3/Accumulator  n_bits=accum_bit_width  overflow=Wrap  operation=Add  scale=1  explicit_period=on  period=-1  rst=on  hasbypass=on  en=off  dbl_ovrd=off  show_param=off  gen_core=on  use_rpm=off
      settings: xl_area=[18 36 0 36 0 0 0]
  Address Control : Subsystem
  Delay2 : xbsIndex_r3/Delay  latency=4  reg_retiming=off  explicit_period=off  period=1  en=off  accept_only_valid=off  init_zero=on  dbl_ovrd=off  show_param=off
      settings: xl_area=[1 1 0 1 0 0 0]
  Down Sample : xbsIndex_r3/Down Sample  sample_ratio=length(coef)/ir  sample_phase="Last Value of Frame  (most efficient)"  latency=1  en=off  dbl_ovrd=off  show_param=off
      settings: xl_area=[18 36 0 0 0 0 0]
  Dual Port RAM : Subsystem
  Mult : xbsIndex_r3/Mult  precision=Full  arith_type="Signed  (2's comp)"  n_bits=8  bin_pt=2  quantization=Truncate  overflow=Wrap  latency=2  explicit_period=off  period=1/(22050*length(coef))  en=off  dbl_ovrd=off  show_param=off  mult_type=Parallel  oversample=2  use_embedded=on  pipeline=on  use_rpm=off  placement_style=Rectangular Shape  gen_core=on
      settings: xl_area=[18 36 0 0 0 1 0]
  Register : xbsIndex_r3/Register  init=0  reg_only_valid=on  explicit_period=on  period=-1  rst=off  en=on  out_en=off  dbl_ovrd=off  show_param=off
      settings: xl_area=[18 36 0 0 0 0 0]
  Dout : Outport
  wires:
  Delay2/1 -> Register/2, Accumulator/2
  Address Control/4(reset) -> Delay2/1
  Dual Port RAM/2(dout_B) -> Mult/2
  Dual Port RAM/1(dout_A) -> Mult/1
  Din/1 -> Dual Port RAM/1(data_A)
  Address Control/3(coef_addr) -> Dual Port RAM/4(addr_B)
  Address Control/2(we) -> Dual Port RAM/3(we_A)
  Address Control/1(data_addr) -> Dual Port RAM/2(addr_A)
  Register/1 -> Down Sample/1
  Accumulator/1 -> Register/1
  Down Sample/1 -> Dout/1
  Mult/1 -> Accumulator/1

== system xrbsDSP_r3/Interpolation Filter ==
  note: The coefficients are arranged in
      | the memory in phase filter order
      | as each phase filter of the polyphase
      | structure is calculated in sequence.
      | The coefficients are pre-arranged by
      | the mask of this block and stored
      | in the appropritate memories
  note: The down sampler is smaller
      | than the initial upsample to
      | achieve the appropriate
      | interpolated rate
  note: The accumulator sums up
      | the partial products from the
      | mult adder tree to form the
      | complete result from each phase
      | filter of the polyphase arms
  note: The 'Adder Tree' subsystem
      | sums the multiplication
      | results after they are
      | caluculated
  note: The 'Multipliers' subsystem
      | employs 4 multiplier to
      | calculate the coefficient
      | and data products.  Data
      | and coefficients are changed
      | to complete the result
  note: As configured, the filter occupies 91 slices, 4 dedicated multiplier, and
      | 4 block memory.  The maximum clock frequency is approximately
      | 199 MHz in a Xilinx xc2vp2-7 part (advanced speeds files 1.69, ISE
      | 5.1.01i software).
  din : Inport
  Accumulator : xbsIndex_r3/Accumulator  n_bits=y_bit_width  overflow=Wrap  operation=Add  scale=1  explicit_period=off  period=1  rst=on  hasbypass=on  en=off  dbl_ovrd=off  show_param=off  gen_core=on  use_rpm=off
      settings: xl_area=[0, 0, 0, 0, 0, 0, 0]
  Adder Tree : Subsystem
  Coef Buffer : Subsystem
  Control : Subsystem
  Data Buffer : Subsystem
  Delay : xbsIndex_r3/Delay  latency=5  reg_retiming=off  explicit_period=off  period=1  en=off  accept_only_valid=off  init_zero=on  dbl_ovrd=off  show_param=off
      settings: xl_area=[0, 0, 0, 0, 0, 0, 0]
  Delay2 : xbsIndex_r3/Delay  latency=1  reg_retiming=off  explicit_period=off  period=1  en=on  accept_only_valid=off  init_zero=on  dbl_ovrd=off  show_param=off
      settings: xl_area=[0, 0, 0, 0, 0, 0, 0]
  Down Sample : xbsIndex_r3/Down Sample  sample_ratio=downsamp_by  sample_phase="Last Value of Frame  (most efficient)"  latency=1  en=off  dbl_ovrd=off  show_param=off
      settings: xl_area=[0, 0, 0, 0, 0, 0, 0]
  Mutlipliers : Subsystem
  Up Sample : xbsIndex_r3/Up Sample  sample_ratio=upsamp_by  copy_samples=on  dbl_ovrd=off  show_param=off
      settings: xl_area=[0, 0, 0, 0, 0, 0, 0]
  Out1 : Outport
  wires:
  Delay2/1 -> Down Sample/1
  Accumulator/1 -> Delay2/1
  Down Sample/1 -> Out1/1
  din/1 -> Up Sample/1
  Adder Tree/1(sum) -> Accumulator/1
  Mutlipliers/4(p3) -> Adder Tree/4(din4)
  Mutlipliers/3(p2) -> Adder Tree/3(din3)
  Mutlipliers/2(p1) -> Adder Tree/2(din2)
  Mutlipliers/1(p0) -> Adder Tree/1(din1)
  Delay/1 -> Delay2/2, Accumulator/2
  Coef Buffer/4(coef3) -> Mutlipliers/8(b3)
  Coef Buffer/3(coef2) -> Mutlipliers/6(b2)
  Coef Buffer/2(coef1) -> Mutlipliers/4(b1)
  Coef Buffer/1(coef0) -> Mutlipliers/2(b0)
  Data Buffer/4(data3) -> Mutlipliers/7(a3)
  Data Buffer/3(data2) -> Mutlipliers/5(a2)
  Data Buffer/2(data1) -> Mutlipliers/3(a1)
  Data Buffer/1(data0) -> Mutlipliers/1(a0)
  Control/4(srl16_we) -> Delay/1
  Control/3(coef_addr) -> Coef Buffer/1(addr)
  Control/2(result) -> Data Buffer/3(shift_en)
  Control/1(data_addr) -> Data Buffer/2(addr)
  Up Sample/1 -> Data Buffer/1(din)
